simulink model "Ambient_Light"  (R2020a)
settings: Solver=VariableStepAuto  StartTime=0.0  StopTime=inf  RelTol=1e-3
undefined symbols (not defined in the file or in its folder): DN, Light, Road_T
libraries: simulink x10
settings Model: Creator=VIJAY BANDEPPA MURGE  LastModifiedBy=VIJAY BANDEPPA MURGE

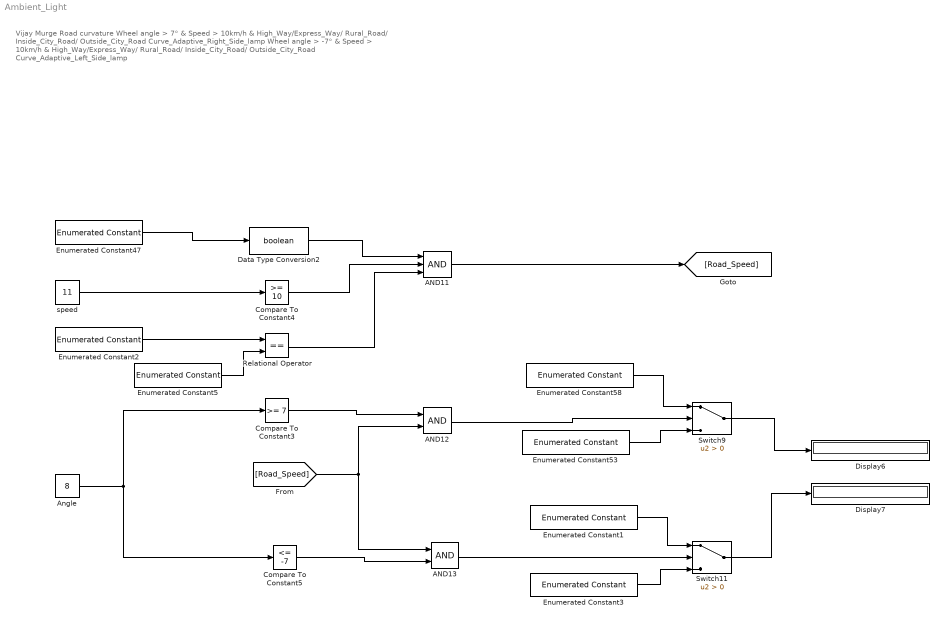
== system Ambient_Light ==
  note: Vijay Murge
      | Road curvature
      | Wheel angle > 7° & Speed > 10km/h & High_Way/Express_Way/ Rural_Road/ Inside_City_Road/ Outside_City_Road
      | Curve_Adaptive_Right_Side_lamp
      |
      | Wheel angle > -7° & Speed > 10km/h & High_Way/Express_Way/ Rural_Road/ Inside_City_Road/ Outside_City_Road
      | Curve_Adaptive_Left_Side_lamp
  AND11 : Logic  Inputs=3  AllPortsSameDT=off  OutDataTypeStr=boolean
  AND12 : Logic  AllPortsSameDT=off  OutDataTypeStr=boolean
  AND13 : Logic  AllPortsSameDT=off  OutDataTypeStr=boolean
  Angle : Constant  Value=8
  Compare To Constant3 : simulink/Logic and Bit Operations/Compare To Constant  relop=>=  const=7  OutDataTypeStr=boolean
  Compare To Constant4 : simulink/Logic and Bit Operations/Compare To Constant  relop=>=  const=10  OutDataTypeStr=boolean
  Compare To Constant5 : simulink/Logic and Bit Operations/Compare To Constant  relop=<=  const=-7  OutDataTypeStr=boolean
  Data Type Conversion2 : DataTypeConversion  OutDataTypeStr=boolean
  Display6 : Display
  Display7 : Display
  Enumerated Constant1 : simulink/Sources/Enumerated Constant  OutDataTypeStr=Enum: Light  Value=Light.L_Ambient_Light_On  SampleTime=inf
  Enumerated Constant2 : simulink/Sources/Enumerated Constant  OutDataTypeStr=Enum: DN  Value=DN.Darkness  SampleTime=inf
  Enumerated Constant3 : simulink/Sources/Enumerated Constant  OutDataTypeStr=Enum: Light  Value=Light.L_Ambient_Light_off  SampleTime=inf
  Enumerated Constant47 : simulink/Sources/Enumerated Constant  OutDataTypeStr=Enum: Road_T  Value=Road_T.High_Way  SampleTime=inf
  Enumerated Constant5 : simulink/Sources/Enumerated Constant  OutDataTypeStr=Enum: DN  Value=DN.Darkness  SampleTime=inf
  Enumerated Constant53 : simulink/Sources/Enumerated Constant  OutDataTypeStr=Enum: Light  Value=Light.R_Ambient_Light_off  SampleTime=inf
  Enumerated Constant58 : simulink/Sources/Enumerated Constant  OutDataTypeStr=Enum: Light  Value=Light.R_Ambient_Light_On  SampleTime=inf
  Relational Operator : RelationalOperator  Operator===  OutDataTypeStr=boolean  RndMeth=Simplest
  Switch11 : Switch  Criteria=u2 > Threshold
  Switch9 : Switch  Criteria=u2 > Threshold
  speed : Constant  Value=11
  wires:
  Enumerated Constant3/1 -> Switch11/3
  Enumerated Constant53/1 -> Switch9/3
  Enumerated Constant5/1 -> Relational Operator/2
  Compare To Constant3/1 -> AND12/1
  [Road_Speed] -> AND13/1, AND12/2
  Enumerated Constant2/1 -> Relational Operator/1
  Data Type Conversion2/1 -> AND11/1
  Enumerated Constant47/1 -> Data Type Conversion2/1
  speed/1 -> Compare To Constant4/1
  Relational Operator/1 -> AND11/3
  Enumerated Constant58/1 -> Switch9/1
  Enumerated Constant1/1 -> Switch11/1
  AND12/1 -> Switch9/2
  Switch11/1 -> Display7/1
  Compare To Constant4/1 -> AND11/2
  AND13/1 -> Switch11/2
  Switch9/1 -> Display6/1
  Compare To Constant5/1 -> AND13/2
  Angle/1 -> Compare To Constant5/1, Compare To Constant3/1
  AND11/1 -> [Road_Speed]
